simulink model "myfirstsimulinkfile_control101"  (R2023a)
settings: Solver=VariableStepAuto  StartTime=0.0  StopTime=endtime  RelTol=1e-3
undefined symbols (not defined in the file): d, Kp, n
settings Model: Creator=Anthony  LastModifiedBy=Anthony Rossiter

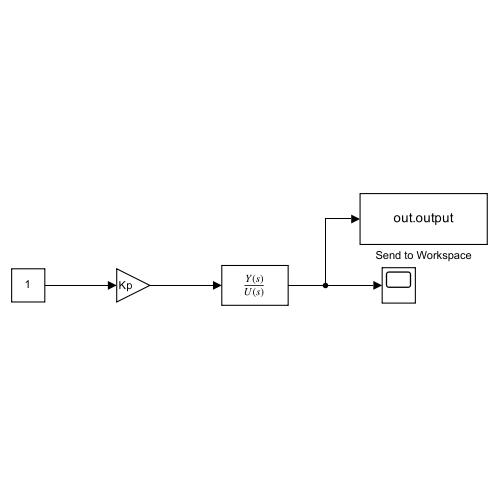
[thumbnail: Simulink's stored preview of the top-level diagram]
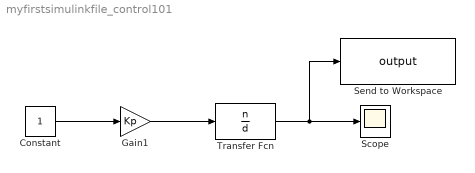
== system myfirstsimulinkfile_control101 ==
  Constant : Constant
  Gain1 : Gain  Gain=Kp
  Scope : Scope
  Send to Workspace : ToWorkspace  VariableName=output  SaveFormat=Structure  SampleTime=-1
  Transfer Fcn : TransferFcn  Numerator=n  Denominator=d
  wires:
  Constant/1 -> Gain1/1
  Gain1/1 -> Transfer Fcn/1
  Transfer Fcn/1 -> Send to Workspace/1, Scope/1
